simulink model "mNextStepTest"  (R2021a)
settings: Solver=FixedStepAuto  StartTime=0.0  StopTime=inf  RelTol=1e-3  EnableMultiTasking=on
libraries: arduinolib x13
settings Model: SILPILModeSetting=veronly  ExtModeTrigDuration=2  Creator=angelo  LastModifiedBy=angelo
settings OptimizationCC: EnhancedBackFolding=on  PassReuseOutputArgsAs=Individual arguments  ZeroExternalMemoryAtStartup=off  ZeroInternalMemoryAtStartup=off  MaxStackSize=64  OptimizeBlockOrder=speed  DifferentSizesBufferReuse=on  OptimizationCustomize=off  EfficientTunableParamExpr=on
settings DebuggingCC: ParameterTunabilityLossMsg=error
settings HardwareCC: ProdBitPerInt=16  ProdBitPerPointer=16  ProdBitPerSizeT=16  ProdBitPerPtrDiffT=16  ProdLargestAtomicFloat=None  ProdWordSize=8  ProdHWDeviceType=Atmel->AVR
settings SFSimCC: MATLABDynamicMemAlloc=off
settings RTWCC: SystemTargetFile=ert.tlc  HardwareBoard=Arduino Mega 2560  TemplateMakefile=ert_default_tmf  Toolchain=Arduino AVR  BuildConfiguration=Faster Runs
settings CodeAppCC: ForceParamTrailComments=on  IgnoreCustomStorageClasses=off  OperatorAnnotations=on  SimulinkDataObjDesc=on  SFDataObjDesc=on  InsertBlockDesc=on
settings ERTTargetCC: SupportContinuousTime=on  SupportVariableSizeSignals=on  ExtModeStaticAllocSize=2048

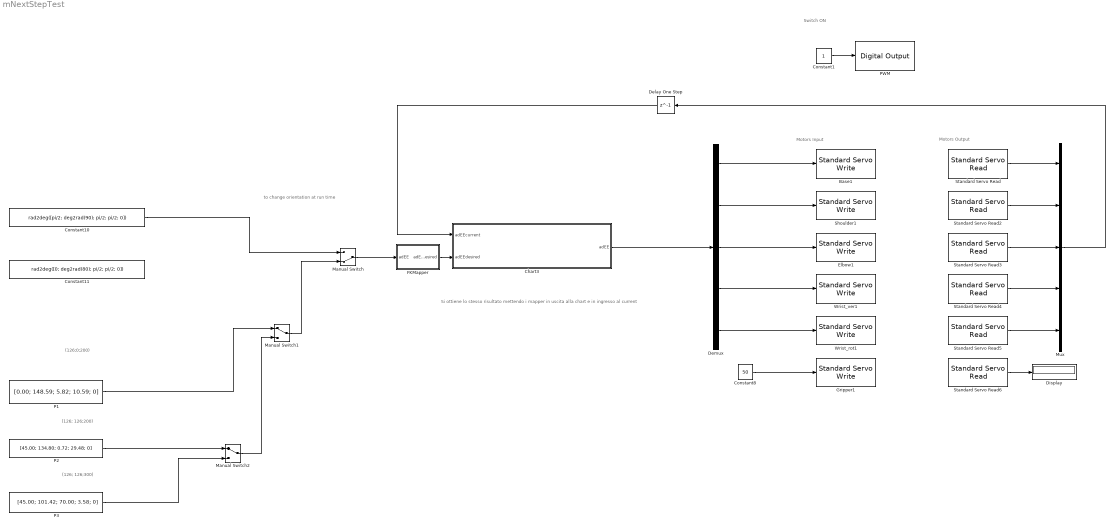
== system mNextStepTest ==
  note: Si ottiene lo stesso risultato mettendo i mapper in uscita alla chart e in ingresso al current
  note: (126;0;200)
  note: to change orientation at run time
  note: Motors Input
  note: Switch ON
  note: (126; 126;200)
  note: (126; 126;300)
  note: Motors Output
  Base1 : arduinolib/Standard Servo Write  pinNumber=11  ServoIndex=0  blockPlatform=ARDUINO
  Chart3 : Stateflow chart  TreatAsAtomicUnit=on  SystemSampleTime=0.02
  Constant1 : Constant
  Constant10 : Constant  Value=rad2deg([pi/2; deg2rad(90); pi/2; pi/2; 0])
  Constant11 : Constant  Value=rad2deg([0; deg2rad(80); pi/2; pi/2; 0])
  Constant8 : Constant  Value=50
  Delay One Step : Delay  DelayLength=1  InitialCondition=[90; 90; 90; 90; 0]
  Demux : Demux  Outputs=5
  Display : Display
  Elbow1 : arduinolib/Standard Servo Write  pinNumber=9  ServoIndex=1  blockPlatform=ARDUINO
  FKMapper : Subsystem
  Gripper1 : arduinolib/Standard Servo Write  pinNumber=3  ServoIndex=2  blockPlatform=ARDUINO
  Manual Switch : ManualSwitch  CurrentSetting=0
  Manual Switch1 : ManualSwitch
  Manual Switch2 : ManualSwitch
  Mux : Mux  Inputs=5
  P1 : Constant  Value=[0.00; 148.59; 5.82; 10.59; 0]
  P2 : Constant  Value=[45.00; 134.80; 0.72; 29.48; 0]
  P3 : Constant  Value=[45.00; 101.42; 70.00; 3.58; 0]
  PWM : arduinolib/Digital Output  pinNumber=12  Direction=output  blockPlatform=arduino
  Shoulder1 : arduinolib/Standard Servo Write  pinNumber=10  ServoIndex=3  blockPlatform=ARDUINO
  Standard Servo Read : arduinolib/Standard Servo Read  pinNumber=11  SampleTime=0.02  ServoIndex=0  blockPlatform=ARDUINO
      settings: SourceProductBaseCode=ARDUINO
  Standard Servo Read2 : arduinolib/Standard Servo Read  pinNumber=10  SampleTime=0.02  ServoIndex=3  blockPlatform=ARDUINO
      settings: SourceProductBaseCode=ARDUINO
  Standard Servo Read3 : arduinolib/Standard Servo Read  pinNumber=9  SampleTime=0.02  ServoIndex=1  blockPlatform=ARDUINO
      settings: SourceProductBaseCode=ARDUINO
  Standard Servo Read4 : arduinolib/Standard Servo Read  pinNumber=6  SampleTime=0.02  ServoIndex=4  blockPlatform=ARDUINO
      settings: SourceProductBaseCode=ARDUINO
  Standard Servo Read5 : arduinolib/Standard Servo Read  pinNumber=5  SampleTime=0.02  ServoIndex=5  blockPlatform=ARDUINO
      settings: SourceProductBaseCode=ARDUINO
  Standard Servo Read6 : arduinolib/Standard Servo Read  pinNumber=3  SampleTime=0.02  ServoIndex=2  blockPlatform=ARDUINO
      settings: SourceProductBaseCode=ARDUINO
  Wrist_rot1 : arduinolib/Standard Servo Write  pinNumber=5  ServoIndex=5  blockPlatform=ARDUINO
  Wrist_ver1 : arduinolib/Standard Servo Write  pinNumber=6  ServoIndex=4  blockPlatform=ARDUINO
  wires:
  Constant8/1 -> Gripper1/1
  Demux/1 -> Base1/1
  Demux/3 -> Elbow1/1
  Demux/5 -> Wrist_rot1/1
  Demux/4 -> Wrist_ver1/1
  Demux/2 -> Shoulder1/1
  Constant1/1 -> PWM/1
  Constant10/1 -> Manual Switch/1
  P1/1 -> Manual Switch1/1
  Manual Switch1/1 -> Manual Switch/2
  P3/1 -> Manual Switch2/2
  P2/1 -> Manual Switch2/1
  Manual Switch2/1 -> Manual Switch1/2
  Standard Servo Read/1 -> Mux/1
  Standard Servo Read2/1 -> Mux/2
  Standard Servo Read3/1 -> Mux/3
  Standard Servo Read4/1 -> Mux/4
  Standard Servo Read5/1 -> Mux/5
  Standard Servo Read6/1 -> Display/1
  Delay One Step/1 -> Chart3/1(adEEcurrent)
  FKMapper/1(adEEdesired) -> Chart3/2(adEEdesired)
  Manual Switch/1 -> FKMapper/1(adEE)
  Chart3/1(adEE) -> Demux/1
  Mux/1 -> Delay One Step/1

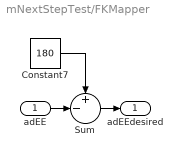
== system mNextStepTest/FKMapper ==
  adEE : Inport
  Constant7 : Constant  Value=180
  Sum : Sum  Inputs=+-|
  adEEdesired : Outport
  wires:
  Sum/1 -> adEEdesired/1
  adEE/1 -> Sum/2
  Constant7/1 -> Sum/1

== stateflow chart mNextStepTest/Chart3 ==
  settings: executeAtInitialization=1
  state First
    during:
    adEE = [
    nextStep(adEEcurrent(1), adEEdesired(1));
    nextStep(adEEcurrent(2), adEEdesired(2));
    nextStep(adEEcurrent(3), adEEdesired(3));
    nextStep(adEEcurrent(4), adEEdesired(4));
    nextStep(adEEcurrent(5), adEEdesired(5)) ];
  (default) -> First
  data: current function_input; desired function_input; v function_output; adEEcurrent input; adEE output; adEEdesired input
  function v = nextStep(current, desired):
    | function v = nextStep(current, desired)
    | if (current < desired)
    |     current = current + 1;
    | end
    | 
    | if (current > desired)
    |     current = current - 1;
    | end
    | 
    | v = current;
    | end
